simulink model "s12_euler_fvm_periodic_step_muscl_minmod_pp_ref"  (R2026a)
settings: Solver=FixedStepDiscrete  StopTime=0
model workspace (MAT data in the model file):
  S12_FVM_CFL = Simulink.Parameter
  S12_FVM_CFL.Value = 0.45
  S12_FVM_CFL.Complexity = 'real'
  S12_FVM_CFL.Dimensions = [1 1]
  S12_FVM_CFL.Description = 'Maximum CFL number'
  S12_FVM_CFL.DataType = 'auto'
  S12_FVM_DtRequest = Simulink.Parameter
  S12_FVM_DtRequest.Value = 0.001
  S12_FVM_DtRequest.Complexity = 'real'
  S12_FVM_DtRequest.Dimensions = [1 1]
  S12_FVM_DtRequest.Description = 'Requested explicit time step'
  S12_FVM_DtRequest.DataType = 'auto'
  S12_FVM_Dx = Simulink.Parameter
  S12_FVM_Dx.Value = 0.01
  S12_FVM_Dx.Complexity = 'real'
  S12_FVM_Dx.Dimensions = [1 1]
  S12_FVM_Dx.Description = 'Uniform cell length'
  S12_FVM_Dx.DataType = 'auto'
  S12_FVM_Gamma = Simulink.Parameter
  S12_FVM_Gamma.Value = 1.4
  S12_FVM_Gamma.Complexity = 'real'
  S12_FVM_Gamma.Dimensions = [1 1]
  S12_FVM_Gamma.Description = 'Heat capacity ratio'
  S12_FVM_Gamma.DataType = 'auto'
  S12_FVM_State = Simulink.Parameter
  S12_FVM_State.Value = [1  1  1  1  0.125  0.125  0.125  0.125; 0  0  0  0  0  0  0  0; 250000  250000  250000  250000  25000  25000  25000  25000]
  S12_FVM_State.Complexity = 'real'
  S12_FVM_State.Dimensions = [3 8]
  S12_FVM_State.Description = 'Rows: density, momentum density, total energy density'
  S12_FVM_State.DataType = 'auto'
  S12_PP_PFloor = Simulink.Parameter
  S12_PP_PFloor.Value = 1e-13
  S12_PP_PFloor.Complexity = 'real'
  S12_PP_PFloor.Dimensions = [1 1]
  S12_PP_PFloor.DataType = 'auto'
  S12_PP_RhoFloor = Simulink.Parameter
  S12_PP_RhoFloor.Value = 1e-13
  S12_PP_RhoFloor.Complexity = 'real'
  S12_PP_RhoFloor.Dimensions = [1 1]
  S12_PP_RhoFloor.DataType = 'auto'
settings Model: Creator=Jovi  LastModifiedBy=Jovi

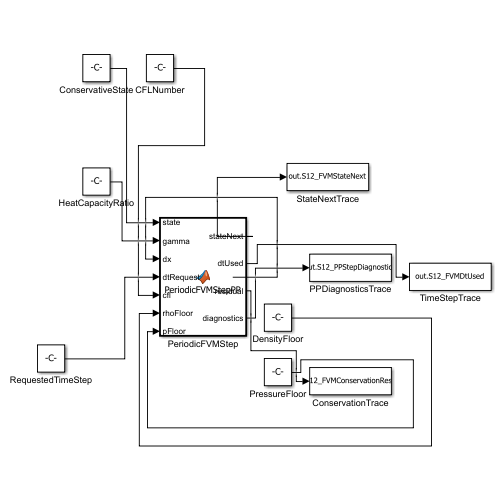
[thumbnail: Simulink's stored preview of the top-level diagram]
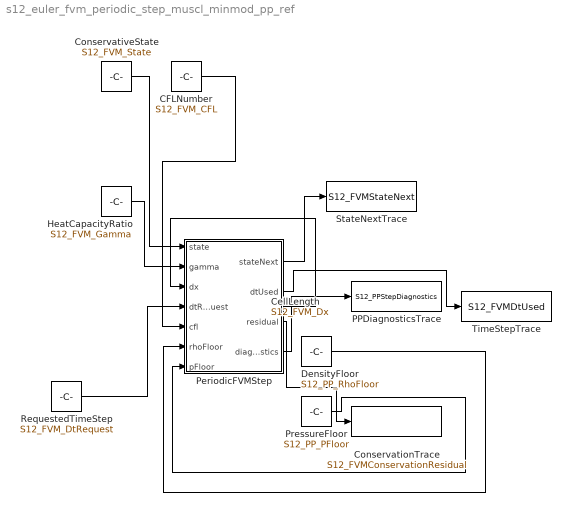
== system s12_euler_fvm_periodic_step_muscl_minmod_pp_ref ==
  CFLNumber : Constant  Value=S12_FVM_CFL
  CellLength : Constant  Value=S12_FVM_Dx
  ConservationTrace : ToWorkspace  VariableName=S12_FVMConservationResidual
      settings: MaxDataPoints=100
  ConservativeState : Constant  Value=S12_FVM_State
  DensityFloor : Constant  Value=S12_PP_RhoFloor
  HeatCapacityRatio : Constant  Value=S12_FVM_Gamma
  PPDiagnosticsTrace : ToWorkspace  VariableName=S12_PPStepDiagnostics
  PeriodicFVMStep : MATLAB Function  TreatAsAtomicUnit=on
  PressureFloor : Constant  Value=S12_PP_PFloor
  RequestedTimeStep : Constant  Value=S12_FVM_DtRequest
  StateNextTrace : ToWorkspace  VariableName=S12_FVMStateNext
      settings: MaxDataPoints=100
  TimeStepTrace : ToWorkspace  VariableName=S12_FVMDtUsed
      settings: MaxDataPoints=100
  wires:
  ConservativeState/1 -> PeriodicFVMStep/1(state)
  HeatCapacityRatio/1 -> PeriodicFVMStep/2(gamma)
  CellLength/1 -> PeriodicFVMStep/3(dx)
  RequestedTimeStep/1 -> PeriodicFVMStep/4(dtRequest)
  CFLNumber/1 -> PeriodicFVMStep/5(cfl)
  PeriodicFVMStep/1(stateNext) -> StateNextTrace/1
  PeriodicFVMStep/2(dtUsed) -> TimeStepTrace/1
  PeriodicFVMStep/3(residual) -> ConservationTrace/1
  DensityFloor/1 -> PeriodicFVMStep/6(rhoFloor)
  PressureFloor/1 -> PeriodicFVMStep/7(pFloor)
  PeriodicFVMStep/4(diagnostics) -> PPDiagnosticsTrace/1

== matlab function s12_euler_fvm_periodic_step_muscl_minmod_pp_ref/PeriodicFVMStep ==
  data: state input; stateNext output; gamma input; dx input; dtRequest input; cfl input; dtUsed output; residual output; rhoFloor input; pFloor input; diagnostics output
function [stateNext,dtUsed,residual,diagnostics] = PeriodicFVMStepPP(state,gamma,dx,dtRequest,cfl,rhoFloor,pFloor)
%#codegen
validateState(state,gamma,rhoFloor,pFloor);
cellCount = size(state,2);
alphaStage = stageAlpha(state,gamma);
dtUsed = min(dtRequest,cfl*dx/alphaStage);
lambda = dtUsed/dx;
[rho,velocity,pressure] = recoverPrimitives(state,gamma);
slopeRho = minmodSlopes(rho);
slopeVelocity = minmodSlopes(velocity);
slopePressure = minmodSlopes(pressure);
leftPrimitive = zeros(3,cellCount);
rightPrimitive = zeros(3,cellCount);
minmodActivationCount = 0;
minmodLimitedCellCount = 0;
reconstructionPPActivationCount = 0;
reconstructionPPLimitedCellCount = 0;
reconstructionPPMinTheta = 1;
minimumReconstructedDensity = inf;
minimumReconstructedPressure = inf;
for cellIndex = 1:cellCount
    leftIndex = mod(cellIndex-2,cellCount)+1;
    rightIndex = mod(cellIndex,cellCount)+1;
    centered = 0.5*[rho(rightIndex)-rho(leftIndex);velocity(rightIndex)-velocity(leftIndex);pressure(rightIndex)-pressure(leftIndex)];
    slopes = [slopeRho(cellIndex);slopeVelocity(cellIndex);slopePressure(cellIndex)];
    limited = abs(slopes-centered) > 32*eps(max([1;abs(slopes);abs(centered)]));
    minmodActivationCount = minmodActivationCount + sum(limited);
    minmodLimitedCellCount = minmodLimitedCellCount + double(any(limited));
    primitive = [rho(cellIndex);velocity(cellIndex);pressure(cellIndex)];
    reconstruction = s12_pp_reconstruct_primitive(primitive,slopes,rhoFloor,pFloor);
    leftPrimitive(:,cellIndex) = reconstruction.left;
    rightPrimitive(:,cellIndex) = reconstruction.right;
    reconstructionPPMinTheta = min(reconstructionPPMinTheta,reconstruction.theta);
    active = reconstruction.theta < 1-32*eps;
    reconstructionPPActivationCount = reconstructionPPActivationCount + double(active);
    reconstructionPPLimitedCellCount = reconstructionPPLimitedCellCount + double(active);
    minimumReconstructedDensity = min(minimumReconstructedDensity,min(reconstruction.left(1),reconstruction.right(1)));
    minimumReconstructedPressure = min(minimumReconstructedPressure,min(reconstruction.left(3),reconstruction.right(3)));
end
interfaceFlux = zeros(3,cellCount);
fluxPPActivationCount = 0;
fluxPPLimitedInterfaceCount = 0;
fluxPPMinTheta = 1;
minimumAnchorDensity = inf;
minimumAnchorPressure = inf;
minimumFinalPartialDensity = inf;
minimumFinalPartialPressure = inf;
maximumFluxCorrectionNorm = 0;
for interfaceIndex = 1:cellCount
    rightIndex = mod(interfaceIndex,cellCount)+1;
    leftState = conservativeFromPrimitives(rightPrimitive(1,interfaceIndex),rightPrimitive(2,interfaceIndex),rightPrimitive(3,interfaceIndex),gamma);
    rightState = conservativeFromPrimitives(leftPrimitive(1,rightIndex),leftPrimitive(2,rightIndex),leftPrimitive(3,rightIndex),gamma);
    highFlux = hllcFlux(leftState,rightState,gamma);
    lowFlux = s12_pp_global_lf_flux(state(:,interfaceIndex),state(:,rightIndex),gamma,alphaStage);
    limitedFlux = s12_pp_limit_interface_flux(state(:,interfaceIndex),state(:,rightIndex),highFlux,lowFlux,lambda,gamma,rhoFloor,pFloor);
    interfaceFlux(:,interfaceIndex) = limitedFlux.flux;
    fluxPPMinTheta = min(fluxPPMinTheta,limitedFlux.theta);
    active = limitedFlux.theta < 1-32*eps;
    fluxPPActivationCount = fluxPPActivationCount + double(active);
    fluxPPLimitedInterfaceCount = fluxPPLimitedInterfaceCount + double(active);
    minimumAnchorDensity = min(minimumAnchorDensity,min(limitedFlux.low_left_partial(1),limitedFlux.low_right_partial(1)));
    minimumAnchorPressure = min(minimumAnchorPressure,min(pressureOf(limitedFlux.low_left_partial,gamma),pressureOf(limitedFlux.low_right_partial,gamma)));
    minimumFinalPartialDensity = min(minimumFinalPartialDensity,min(limitedFlux.left_partial(1),limitedFlux.right_partial(1)));
    minimumFinalPartialPressure = min(minimumFinalPartialPressure,min(pressureOf(limitedFlux.left_partial,gamma),pressureOf(limitedFlux.right_partial,gamma)));
    maximumFluxCorrectionNorm = max(maximumFluxCorrectionNorm,limitedFlux.correction_norm);
end
stateNext = zeros(size(state));
for cellIndex = 1:cellCount
    leftInterface = mod(cellIndex-2,cellCount)+1;
    stateNext(:,cellIndex) = state(:,cellIndex)-lambda*(interfaceFlux(:,cellIndex)-interfaceFlux(:,leftInterface));
end
validateState(stateNext,gamma,rhoFloor,pFloor);
residual = sum(stateNext-state,2).';
diagnostics = [minmodActivationCount,minmodLimitedCellCount,cellCount,reconstructionPPActivationCount,reconstructionPPLimitedCellCount,reconstructionPPMinTheta,minimumReconstructedDensity,minimumReconstructedPressure,0,fluxPPActivationCount,fluxPPLimitedInterfaceCount,cellCount,fluxPPMinTheta,minimumAnchorDensity,minimumAnchorPressure,minimumFinalPartialDensity,minimumFinalPartialPressure,alphaStage,maximumFluxCorrectionNorm,0];
end

function alpha = stageAlpha(state,gamma)
[rho,velocity,pressure] = recoverPrimitives(state,gamma);
alpha = max(abs(velocity)+sqrt(gamma*pressure./rho));
end

function validateState(state,gamma,rhoFloor,pFloor)
[rho,~,pressure] = recoverPrimitives(state,gamma);
if any(~isfinite(state(:))) || any(rho < rhoFloor) || any(pressure < pFloor)
    error('S12:Positivity:InvalidStage','A PP stage violated the configured floors.');
end
end

function [rho,velocity,pressure] = recoverPrimitives(state,gamma)
rho = state(1,:);
velocity = state(2,:)./rho;
pressure = (gamma-1)*(state(3,:)-0.5*rho.*velocity.^2);
end

function value = pressureOf(state,gamma)
rho = state(1);
velocity = state(2)/rho;
value = (gamma-1)*(state(3)-0.5*rho*velocity^2);
end

function state = conservativeFromPrimitives(rho,velocity,pressure,gamma)
state = [rho;rho*velocity;pressure/(gamma-1)+0.5*rho*velocity^2];
end

function slopes = minmodSlopes(values)
cellCount = numel(values);
slopes = zeros(size(values));
for cellIndex = 1:cellCount
    leftIndex = mod(cellIndex-2,cellCount)+1;
    rightIndex = mod(cellIndex,cellCount)+1;
    slopes(cellIndex) = minmod(values(cellIndex)-values(leftIndex),values(rightIndex)-values(cellIndex));
end
end

function value = minmod(leftDelta,rightDelta)
if leftDelta*rightDelta <= 0
    value = 0;
elseif abs(leftDelta) <= abs(rightDelta)
    value = leftDelta;
else
    value = rightDelta;
end
end

function flux = hllcFlux(stateL,stateR,gamma)
rhoL = stateL(1); rhoR = stateR(1);
uL = stateL(2)/rhoL; uR = stateR(2)/rhoR;
energyL = stateL(3); energyR = stateR(3);
pL = (gamma-1)*(energyL-0.5*rhoL*uL*uL);
pR = (gamma-1)*(energyR-0.5*rhoR*uR*uR);
soundL = sqrt(gamma*pL/rhoL); soundR = sqrt(gamma*pR/rhoR);
sL = min(uL-soundL,uR-soundR); sR = max(uL+soundL,uR+soundR);
sM = (pR-pL+rhoL*uL*(sL-uL)-rhoR*uR*(sR-uR))/(rhoL*(sL-uL)-rhoR*(sR-uR));
fluxL = [rhoL*uL;rhoL*uL*uL+pL;uL*(energyL+pL)];
fluxR = [rhoR*uR;rhoR*uR*uR+pR;uR*(energyR+pR)];
if sL >= 0
    flux = fluxL;
elseif sM >= 0
    rhoStarL = rhoL*(sL-uL)/(sL-sM);
    energyStarL = rhoStarL*(energyL/rhoL+(sM-uL)*(sM+pL/(rhoL*(sL-uL))));
    flux = fluxL+sL*([rhoStarL;rhoStarL*sM;energyStarL]-stateL);
elseif sR > 0
    rhoStarR = rhoR*(sR-uR)/(sR-sM);
    energyStarR = rhoStarR*(energyR/rhoR+(sM-uR)*(sM+pR/(rhoR*(sR-uR))));
    flux = fluxR+sR*([rhoStarR;rhoStarR*sM;energyStarR]-stateR);
else
    flux = fluxR;
end
end
